simulink model "dp_observer_unit_test"  (R2016b)
settings: Solver=ode3  StartTime=0.0  StopTime=100  FixedStep=0.01  RelTol=1e-3  EnableMultiTasking=on
values from neighbouring files (symbols this model uses):
  K2 = diag([200,50,3])    [Input_v3.m]    (also in inputDPgains.m = [1 0 0; 0 1 0; 0 0 1])
undefined symbols (not defined in the file or in its folder): L1, L2, L3
libraries: simulink x3
settings Model: Creator=MCLab  LastModifiedBy=ssp
settings DataIOCC: LimitDataPoints=on  SaveFormat=Array
settings OptimizationCC: LifeSpan=inf
settings DebuggingCC: SFUnexpectedBacktrackingDiag=warning  SFNoUnconditionalDefaultTransitionDiag=warning  SFExecutionAtInitializationDiag=none
settings HardwareCC: ProdBitPerPointer=32  ProdBitPerSizeT=32  ProdBitPerPtrDiffT=32  ProdLargestAtomicFloat=None  ProdIntDivRoundTo=Undefined  ProdEndianess=Unspecified  ProdWordSize=32  ProdHWDeviceType=32-bit Generic
settings ModelReferenceCC: PropagateSignalLabelsOutOfModel=off
settings GRTTargetCC: TargetLangStandard=C89/C90 (ANSI)  GeneratePreprocessorConditionals=Disable all
settings ConfigComp: CovMetricSettings=dw  CovHtmlReporting=on  CovSaveCumulativeToWorkspaceVar=on  CovSaveSingleToWorkspaceVar=on  CovExternalEMLEnable=off

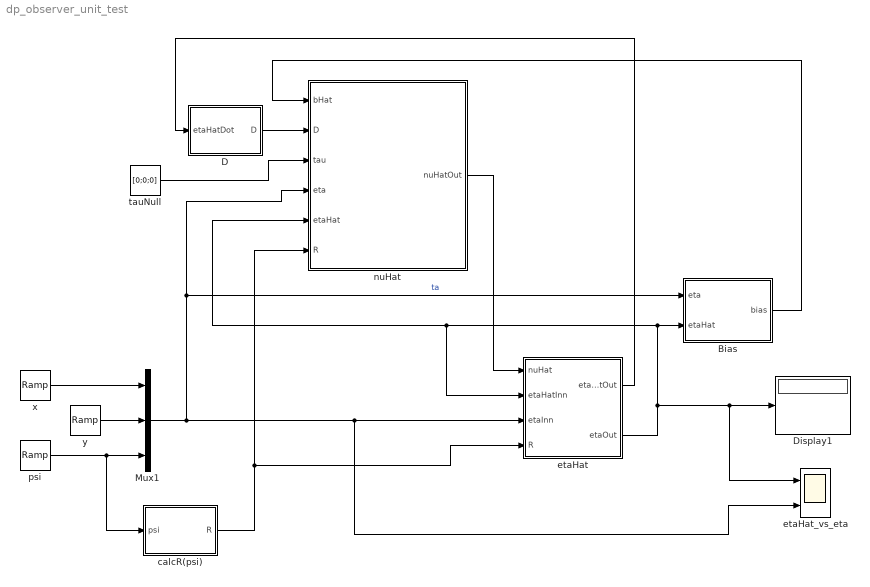
== system dp_observer_unit_test ==
  Bias : Subsystem
  D : MATLAB Function  TreatAsAtomicUnit=on
  Display1 : Display
  Mux1 : Mux  Inputs=3
  "calcR(psi) " : MATLAB Function  TreatAsAtomicUnit=on
  etaHat : Subsystem
  etaHat_vs_eta : Scope  NumInputPorts=2
  nuHat : Subsystem
  psi : simulink/Sources/Ramp  slope=0.01  start=5  X0=0
  "tauNull " : Constant  Value=[0;0;0]
  x : simulink/Sources/Ramp  slope=0.05  start=.1  X0=0
  y : simulink/Sources/Ramp  slope=0.06  start=10  X0=0
  wires:
  y/1 -> Mux1/2
  psi/1 -> "calcR(psi) "/1(psi), Mux1/3
  Mux1/1 -> etaHat_vs_eta/2, etaHat/3(etaInn), nuHat/4(eta), Bias/1(eta)  "ta"
  "calcR(psi) "/1(R) -> nuHat/6(R), etaHat/4(R)
  x/1 -> Mux1/1
  etaHat/2(etaOut) -> nuHat/5(etaHat), etaHat/2(etaHatInn), Bias/2(etaHat), Display1/1, etaHat_vs_eta/1
  etaHat/1(etaHatOut) -> D/1(etaHatDot)
  D/1(D) -> nuHat/2(D)
  Bias/1(bias) -> nuHat/1(bHat)
  "tauNull "/1 -> nuHat/3(tau)
  nuHat/1(nuHatOut) -> etaHat/1(nuHat)

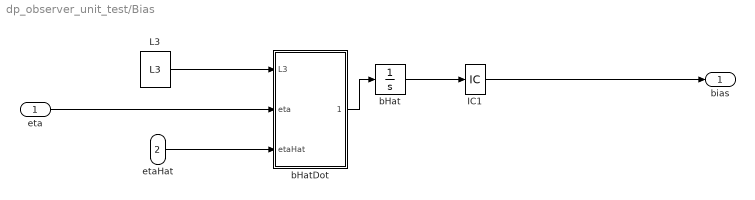
== system dp_observer_unit_test/Bias ==
  eta : Inport
  etaHat : Inport  Port=2
  IC1 : InitialCondition  Value=[0;0;0]
  L3 : Constant  Value=L3
  bHat : Integrator
  bHatDot : MATLAB Function  TreatAsAtomicUnit=on
  bias : Outport
  wires:
  bHatDot/1(bHatDot) -> bHat/1
  bHat/1 -> IC1/1
  eta/1 -> bHatDot/2(eta)
  etaHat/1 -> bHatDot/3(etaHat)
  L3/1 -> bHatDot/1(L3)
  IC1/1 -> bias/1

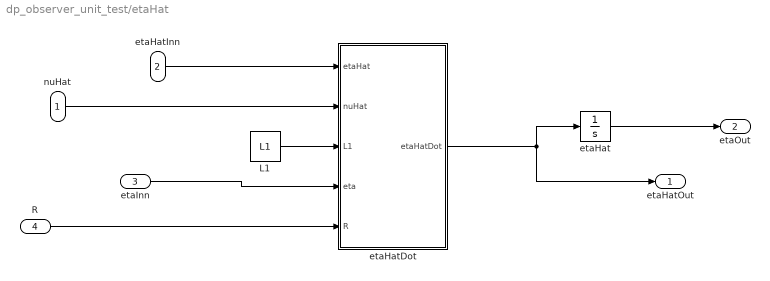
== system dp_observer_unit_test/etaHat ==
  nuHat : Inport
  etaHatInn : Inport  Port=2
  etaInn : Inport  Port=3
  R : Inport  Port=4
  L1 : Constant  Value=L1
  etaHat : Integrator
  etaHatDot : MATLAB Function  TreatAsAtomicUnit=on
  etaHatOut : Outport
  etaOut : Outport  Port=2
  wires:
  etaHat/1 -> etaOut/1
  etaHatDot/1(etaHatDot) -> etaHat/1, etaHatOut/1
  L1/1 -> etaHatDot/3(L1)
  R/1 -> etaHatDot/5(R)
  nuHat/1 -> etaHatDot/2(nuHat)
  etaInn/1 -> etaHatDot/4(eta)
  etaHatInn/1 -> etaHatDot/1(etaHat)

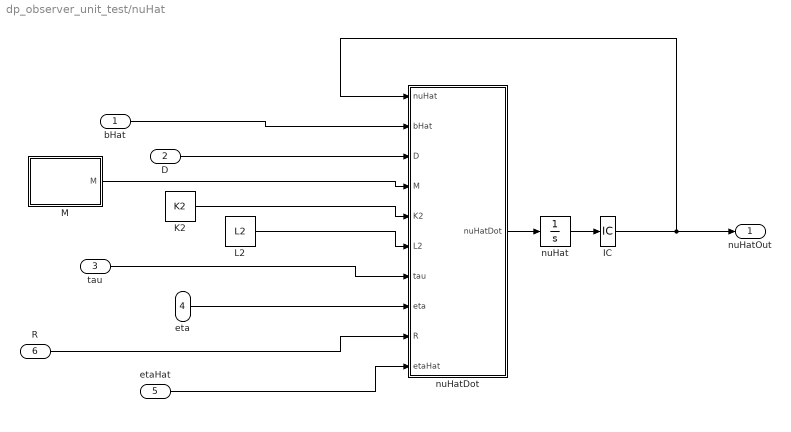
== system dp_observer_unit_test/nuHat ==
  bHat : Inport
  D : Inport  Port=2
  tau : Inport  Port=3
  eta : Inport  Port=4
  etaHat : Inport  Port=5
  R : Inport  Port=6
  IC : InitialCondition  Value=[0;0;0]
  K2 : Constant  Value=K2
  "L2 " : Constant  Value=L2
  M : MATLAB Function  TreatAsAtomicUnit=on
  nuHat : Integrator
  nuHatDot : MATLAB Function  TreatAsAtomicUnit=on
  nuHatOut : Outport
  wires:
  K2/1 -> nuHatDot/5(K2)
  nuHat/1 -> IC/1
  tau/1 -> nuHatDot/7(tau)
  bHat/1 -> nuHatDot/2(bHat)
  M/1(M) -> nuHatDot/4(M)
  IC/1 -> nuHatDot/1(nuHat), nuHatOut/1
  etaHat/1 -> nuHatDot/10(etaHat)
  R/1 -> nuHatDot/9(R)
  eta/1 -> nuHatDot/8(eta)
  nuHatDot/1(nuHatDot) -> nuHat/1
  D/1 -> nuHatDot/3(D)
  "L2 "/1 -> nuHatDot/6(L2)

== matlab function dp_observer_unit_test/etaHat/etaHatDot ==
  data: etaHat input; nuHat input; L1 input; eta input; R input; etaHatDot output
function etaHatDot = fcn(etaHat,nuHat,L1,eta,R)

%etaHatDot=zeros(3,1);
etaHatDot=R*nuHat+L1*(eta-etaHat);

end

== matlab function dp_observer_unit_test/calcR(psi)  ==
  data: psi input; R output
function R = fcn(psi)

R=[cos(psi) -sin(psi) 0; sin(psi) cos(psi) 0; 0 0 1];

end

== matlab function dp_observer_unit_test/nuHat/nuHatDot ==
  data: nuHat input; bHat input; D input; M input; K2 input; L2 input; tau input; eta input; R input; etaHat input; nuHatDot output
function nuHatDot = fcn(nuHat,bHat,D,M,K2,L2,tau,eta,R,etaHat)

nuHatDot=inv(M)*(-D*nuHat+transpose(R)*bHat+tau+K2*transpose(R)*L2*(eta-etaHat));
end

== matlab function dp_observer_unit_test/nuHat/M ==
  data: M output
function M = void

m=14.79;
M=[m+2 0 0; 0 m+10 m*0.0375; 0 m*0.0375 1.76+1];

end

== matlab function dp_observer_unit_test/D ==
  data: D output; etaHatDot input
function D = fcn(etaHatDot)

u=0; %etaHatDot(1,1);
v=0; %etaHatDot(2,2);
r=0; %etaHatDot(3,3);

Xu=-0.6555;
Xuu=0.3545;
Xuuu=-3.787;
Yv=-1.33;
Yvv=-2.776;
Yvvv=-64.91;
Yr=-7.25;
Yrr=-3.45;
Yrrr=0;
Yrv=-0.805;
Yvr=-0.845;
Nv=0;
Nvv=-0.2088;
Nvvv=0;
Nr=-1.9;
Nrr=-0.75;
Nrrr=0;
Nrv=0.13;
Nvr=0.08;

d11=-Xu-Xuu*abs(u)-Xuuu*u^2;
d22=-Yv-Yvv*abs(v)-Yvvv*v^2-Yrv*abs(r);
d23=-Yr-Yvr*abs(v)-Yrr*abs(r)-Yrrr*r^2;
d32=-Nv-Nvv*abs(v)-Nvvv*v^2-Nrv*abs(r);
d33=-Nr-Nvr*abs(v)-Nrr*abs(r)-Nrrr*r^2;

D=[d11 0 0; 0 d22 d23; 0 d32 d33];

end

== matlab function dp_observer_unit_test/Bias/bHatDot ==
  data: bHatDot output; L3 input; eta input; etaHat input
function bHatDot = fcn(L3,eta,etaHat)

bHatDot=L3*(eta-etaHat);

end
